simulink model "Copy_of_MPC_control"  (R2018a)
settings: Solver=FixedStepAuto  StartTime=0  StopTime=Tend  FixedStep=0.001  RelTol=5e-3
model workspace (MAT data in the model file):
  A_mu = 10
  B_reff = 8.386
  Cz = 7766.25
  DCT_Param : struct (value not decoded)
  D_reff = 0.25826
  Downshift_Speeds = [9.5625 12.9375 16.3125 19.6875 23.0625 26.4375 29.8125 33.1875 36.5625 39.9375 43.3125 46.6875 ... (28 elements, 4x7)]
  Pedal_Positions = [0.1 0.4 0.5 0.9]
  SUS : struct (value not decoded)
  Upshift_Speeds = [12.9375 16.3125 19.6875 33 26.4375 29.8125 33.1875 52.5 39.9375 43.3125 46.6875 77.25 ... (28 elements, 4x7)]
  VEH : struct (value not decoded)
  V_o = 16.7
  V_xlow = 1
  WH : struct (value not decoded)
  a = 1.4
  alpha_max = 1.5
  alpha_min = -1.5
  b = 1.8
  c_zo = 209651
  epsilon = 0.1
  h = 0.134
  path : struct (value not decoded)
  pio = 220000
  q_Fcx = 0
  q_Fz2 = 15.4
  q_Fzy = 0
  q_reo = 0.9974
  q_sx1 = -0.007764
  q_sx10 = 0.2824
  q_sx11 = 5.349
  q_sx12 = 0
  q_sx13 = 0
  q_sx14 = 0
  q_sx2 = 1.1915
  q_sx3 = 0.013948
  q_sx4 = 4.912
  q_sx5 = 1.02
  q_sx6 = 22.83
  q_sx7 = 0.7104
  q_sx8 = -0.023393
  q_sx9 = 0.6581
  q_sy1 = 0.00702
  q_sy2 = 0
  q_sy3 = 0.001515
  q_sy4 = 8.514e-05
  q_sy5 = 0
  q_sy6 = 0
  q_sy7 = 0.9008
  q_sy8 = -0.4089
  q_v1 = 0.0007742
  q_v2 = 0.04667
  r_Bx1 = 12.531
  r_Bx2 = 9.532
  r_Bx3 = 0
  r_By1 = 10.615
  r_By2 = 7.705
  r_By3 = 3.433e-06
  r_By4 = 0
  r_Cx1 = 1.019
  r_Cy1 = 1.0585
  r_Ex1 = -0.4487
  r_Ex2 = -0.4726
  r_Ey1 = 0.3132
  r_Ey2 = 7.63e-06
  r_Hx1 = 0.0002374
  r_Hy1 = 0.011646
  r_Hy2 = 7.63e-06
  r_Vy1 = 0.05654
  r_Vy2 = 7.63e-06
  r_Vy3 = 0
  r_Vy4 = 99.9
  r_Vy5 = 2
  r_Vy6 = 15.814
  r_o = 0.3135
  vehWidth = 2
  w = 1
symbols that are objects in the model workspace (value not decoded): VEH
undefined symbols (not defined in the file): C_Brake, C_Final, C_Front, C_Front_1, C_Front_2, C_Middle, C_out_Brake, C_out_Final, C_out_Front, C_out_Front_1, C_out_Front_2, C_out_Middle, Co, Cok_Brake, Cok_Final, Cok_Front_1, Cok_Front_2, Cok_Middle, Cso, D_out_Brake, D_out_Final, D_out_Front, D_out_Front_1, D_out_Front_2, D_out_Middle, Earlytochange, Earlytochange2, F, F_Brake, F_Final, F_Front, F_Front_1, F_Front_2, F_Middle, Fs, G_Brake, G_Final, G_Front_1, G_Front_2, G_Middle, G_sys_Brake, G_sys_Final, G_sys_Front, G_sys_Front_1, G_sys_Front_2, G_sys_Middle, Gd, Gd_Brake, Gd_Final, Gd_Front, Gd_Front_1, Gd_Front_2, Gd_Middle, Go, Gsd, Gso, H_Brake, H_Final, H_Front_1, H_Front_2 ... (+60)
libraries: simulink x10, sim3dlib x4, autolibutils x2, vehdynlibviscommon x2
(part 6 of 8)

== system Copy_of_MPC_control/all_system/Middle Observer2/Subsystem/Mpc_Simulator_Middle ==
  Vup : Inport  SampleTime=Ts  LockScale=on
  Yup : Inport  Port=2  SampleTime=Ts  LockScale=on
  Rs_V : Inport  Port=3  SampleTime=Ts  LockScale=on
  Rs : Inport  Port=4  SampleTime=Ts  LockScale=on
  Xh_sim : Inport  Port=5
  Clock : Clock
  Constant1 : Constant  Value=M  VectorParams1D=off  SampleTime=-1
  Constant2 : Constant  Value=Np  SampleTime=-1
  Constant3 : Constant  Value=Upd_flag  VectorParams1D=off  SampleTime=-1
  Constant4 : Constant  Value=Qc  VectorParams1D=off  SampleTime=-1
  Constant5 : Constant  Value=phi_Middle  VectorParams1D=off  SampleTime=-1
  Constant6 : Constant  Value=JE_Middle  VectorParams1D=off  SampleTime=-1
  Constant7 : Constant  Value=Upd_end  VectorParams1D=off  SampleTime=-1
  Constant8 : Constant  Value=Timetochange  VectorParams1D=off  SampleTime=-1
  F_Middle : Gain  Gain=F_Middle  Multiplication=Matrix(K*u) (u vector)
  MATLAB Function : MATLAB Function  TreatAsAtomicUnit=on  SystemSampleTime=Ts
  Unit Delay : UnitDelay  InitialCondition=[0;0]  SampleTime=Ts
  U : Outport
  Ref : Outport  Port=2
  wires:
  Unit Delay/1 -> MATLAB Function/15(u)
  MATLAB Function/2(U) -> Unit Delay/1, U/1
  MATLAB Function/1(Ref) -> Ref/1
  Xh_sim/1 -> F_Middle/1
  Constant4/1 -> MATLAB Function/7(Qc)
  Constant5/1 -> MATLAB Function/6(phi)
  Constant6/1 -> MATLAB Function/3(JE)
  Constant2/1 -> MATLAB Function/5(Np)
  Rs_V/1 -> MATLAB Function/12(Rs_V)
  Yup/1 -> MATLAB Function/9(Yup)
  Constant1/1 -> MATLAB Function/4(M)
  Clock/1 -> MATLAB Function/13(Tsim)
  F_Middle/1 -> MATLAB Function/8(Fxh)
  Vup/1 -> MATLAB Function/10(Vup)
  Rs/1 -> MATLAB Function/11(Rs)
  Constant3/1 -> MATLAB Function/1(Upd_flag)
  Constant7/1 -> MATLAB Function/14(Upd_end)
  Constant8/1 -> MATLAB Function/2(Timetochange)

== system Copy_of_MPC_control/all_system/Middle Observer2/Subsystem/Pose updete k ==
  XYplot_sim : Inport
  Velocity_sim : Inport  Port=2
  Heading_sim : Inport  Port=3
  Clock : Clock
  From Workspace : FromWorkspace  VariableName=Rs_V_now  SampleTime=Ts
  From Workspace1 : FromWorkspace  VariableName=Rs_Y_now  SampleTime=Ts
  From Workspace2 : FromWorkspace  VariableName=XYplot_X  SampleTime=Ts
  From Workspace3 : FromWorkspace  VariableName=XYplot_Y  SampleTime=Ts
  Mux : Mux  Inputs=2
  Reshape : Reshape  OutputDimensionality=Customize  OutputDimensions=[pick_num,2]
  Trajectroy : Constant  Value=XYplot  VectorParams1D=off  SampleTime=-1
  Unit Delay{,1..3} (4 alike) : UnitDelay  SampleTime=Ts
  Update : MATLAB Function  TreatAsAtomicUnit=on  SystemSampleTime=Ts
      settings: RTWFcnNameOpts=Use subsystem name
  Velocity_updated : Outport
  Heading_updated : Outport  Port=2
  wires:
  XYplot_sim/1 -> Update/5(XYplot_sim), Unit Delay3/1
  Heading_sim/1 -> Unit Delay2/1, Update/9(Heading_sim)
  Clock/1 -> Update/11(Tsim)
  Velocity_sim/1 -> Update/7(Velocity_sim), Unit Delay1/1
  Update/2(Heading_updated) -> Heading_updated/1
  Update/1(Velocity_updated) -> Velocity_updated/1
  From Workspace/1 -> Update/1(Rs_V_now)
  Update/3(Heading_end) -> Unit Delay/1
  Unit Delay/1 -> Update/12(Last_Heading_end)
  From Workspace1/1 -> Update/2(Rs_Y_now)
  Unit Delay1/1 -> Update/8(Last_Velocity_sim)
  Unit Delay2/1 -> Update/10(Last_Heading_sim)
  Unit Delay3/1 -> Update/6(Last_XYplot_sim)
  Mux/1 -> Reshape/1
  From Workspace2/1 -> Mux/1
  From Workspace3/1 -> Mux/2
  Trajectroy/1 -> Update/3(XYline)
  Reshape/1 -> Update/4(XYplot)

== system Copy_of_MPC_control/all_system/Middle Observer2/Subsystem/VH2P ==
  Velocities : Inport
  HeadingAngles : Inport  Port=2
  Initial position : Inport  Port=3
  Iintial Velocities : Inport  Port=4
  Iintial HeadingAngles : Inport  Port=5
  Tsim : Inport  Port=6
  LastTsim : Inport  Port=7
  Resettable Delay : Delay  DelayLength=1  InitialConditionSource=Input port  SampleTime=Ts
      settings: InputPortMap=u0,p4
  Resettable Delay1 : Delay  DelayLength=1  InitialConditionSource=Input port  SampleTime=Ts
      settings: InputPortMap=u0,p4
  Resettable Delay2 : Delay  DelayLength=1  InitialConditionSource=Input port  SampleTime=Ts
      settings: InputPortMap=u0,p4
  YV2P : MATLAB Function  TreatAsAtomicUnit=on  SystemSampleTime=Ts
  Position : Outport
  wires:
  YV2P/1(Position) -> Resettable Delay/1, Position/1
  LastTsim/1 -> YV2P/6(LastTsim)
  Velocities/1 -> Resettable Delay1/1, YV2P/1(Velocity)
  Resettable Delay1/1 -> YV2P/3(LastVelocity)
  HeadingAngles/1 -> YV2P/2(Yaw), Resettable Delay2/1
  Resettable Delay2/1 -> YV2P/4(LastYaw)
  Resettable Delay/1 -> YV2P/7(Lastpostion)
  Initial position/1 -> Resettable Delay/2
  Iintial Velocities/1 -> Resettable Delay1/2
  Iintial HeadingAngles/1 -> Resettable Delay2/2
  Tsim/1 -> YV2P/5(Tsim)

== system Copy_of_MPC_control/all_system/Middle Observer2/Subsystem/YV_update_Np ==
  XY_sim : Inport
  Velocity_sim : Inport  Port=2
  Heading_sim : Inport  Port=3
  From Workspace1 : FromWorkspace  VariableName=T_sim  SampleTime=Ts
  From Workspace3 : FromWorkspace  VariableName=XY_Ref_Upd  SampleTime=Ts
  MATLAB Function2 : MATLAB Function  TreatAsAtomicUnit=on  SystemSampleTime=Ts
  Unit Delay1 : UnitDelay  SampleTime=Ts
  Unit Delay4 : UnitDelay  SampleTime=Ts
  Unit Delay5 : UnitDelay  SampleTime=Ts
  Velocity : Outport
  Heading angle : Outport  Port=2
  wires:
  MATLAB Function2/1(Velocity_updated) -> Velocity/1
  From Workspace3/1 -> MATLAB Function2/1(XY_ref)
  MATLAB Function2/2(Heading_updated) -> Heading angle/1
  From Workspace1/1 -> MATLAB Function2/8(Tsim)
  XY_sim/1 -> Unit Delay1/1, MATLAB Function2/2(XY_sim)
  Velocity_sim/1 -> MATLAB Function2/4(Velocity_sim), Unit Delay5/1
  Heading_sim/1 -> MATLAB Function2/6(Yaw_sim), Unit Delay4/1
  Unit Delay1/1 -> MATLAB Function2/3(LastXY_sim)
  Unit Delay5/1 -> MATLAB Function2/5(LastVelocity_sim)
  Unit Delay4/1 -> MATLAB Function2/7(LastYaw_sim)

== system Copy_of_MPC_control/all_system/Middle_simulator1/VH2P/Trigger ==
  Clock9 : Clock
  Constant1 : Constant  Value=Timetochange
  Trigger : MATLAB Function  TreatAsAtomicUnit=on
  Trig : Outport
  wires:
  Constant1/1 -> Trigger/2(Timetochange)
  Clock9/1 -> Trigger/1(timing)
  Trigger/1(Trigger) -> Trig/1

== system Copy_of_MPC_control/all_system/Visualization1/3D Engine/3D Engine ==
  VehFdbk : Inport
  3D Body Offset : Constant  Value=single(0.0112)  OutDataTypeStr=single
  Add1 : Sum  Inputs=-+
  Add3 : Sum  Inputs=-+-
  Bus Selector : BusSelector  OutputSignals=Body.X,Body.Y,Body.Z,Body.phi,Body.theta,Body.psi
  Bus Selector2 : BusSelector  OutputSignals=Wheels.zAxle,Wheels.omega,Driveline.WhlAng
  Bus Selector3 : BusSelector  OutputSignals=Body.ZHP
  Constant1 : Constant  Value=zeros(4,1)  OutDataTypeStr=single
  Constant2 : Constant  Value=0  OutDataTypeStr=single
  Constant8 : Constant  Value=h
  Data Type Conversion{1,4..10,12} (9 alike) : DataTypeConversion  OutDataTypeStr=single
  Demux{,1..3} (4 alike) : Demux
  Integrator : Integrator  WrapState=on  WrappedStateUpperValue=2*pi  WrappedStateLowerValue=0  ZeroCross=off
  Part Rotation Concatenation : Subsystem
  Part Translation Concatenation : Subsystem
  Rate Transition : RateTransition  OutPortSampleTime=dt3D
  Scale : Subsystem
  Simulation 3D Engine 1 : sim3dlib/Simulation 3D Config  Priority=1  ProjectFormat=Executable  ProjectName=VehicleSimulation.exe  SceneDesc=Straight road  OpVisEn=off  Ts=dt3D
      settings: AttributesFormatString=Priority: %<Priority>
  Unary Minus : UnaryMinus
  Vehicle Actor Transform Set : sim3dlib/Simulation 3D Actor Transform Set  ActorTag=SimulinkVehicle1  ActorType=Passenger vehicle  PassVehMesh=Muscle car  VehColor=Red  NumberOfParts=5  CustNumOfParts=3  Translation=[0 0 1; 0 0 0; 0 0 0; 0 0 0; 0 0 0]  Rotation=[0 0 0; 0 0 0; 0 0 0; 0 0 0; 0 0 0]  Scale=[1 1 1; 1 1 1; 1 1 1; 1 1 1; 1 1 1]  Ts=dt3D
  wires:
  Unary Minus/1 -> Integrator/1
  Bus Selector3/1 -> Add3/2  "<ZHP>"
  Add3/1 -> Data Type Conversion12/1
  Bus Selector2/1 -> Add3/3  "<zAxle>"
  Constant8/1 -> Add3/1
  Rate Transition/1 -> Bus Selector/1, Bus Selector3/1, Bus Selector2/1
  Scale/1(ScaleOut) -> Vehicle Actor Transform Set/3
  Demux/4 -> Part Rotation Concatenation/7(WheelRearRight Ptich)
  Demux/3 -> Part Rotation Concatenation/6(WheelRearLeft Pitch)
  Demux/2 -> Part Rotation Concatenation/5(WheelFrontRight Pitch)
  Demux/1 -> Part Rotation Concatenation/4(WheelFrontLeft Pitch)
  Constant1/1 -> Demux2/1
  Bus Selector/4 -> Data Type Conversion7/1  "<phi>"
  Data Type Conversion6/1 -> Add1/1
  Part Rotation Concatenation/1(ConcatOut) -> Vehicle Actor Transform Set/2
  Part Translation Concatenation/1(ConcatOut) -> Vehicle Actor Transform Set/1
  Data Type Conversion12/1 -> Demux3/1
  Demux3/4 -> Part Translation Concatenation/15(WheelRearRightZ)
  Demux3/3 -> Part Translation Concatenation/14(WheelRearLeftZ)
  Demux3/1 -> Part Translation Concatenation/12(WheelFrontLeftZ)
  Demux3/2 -> Part Translation Concatenation/13(WheelFrontRightZ)
  VehFdbk/1 -> Rate Transition/1
  Add1/1 -> Part Translation Concatenation/3(BodyZ)
  3D Body Offset/1 -> Add1/2
  Demux1/4 -> Part Rotation Concatenation/15(WheelRearRight Yaw)
  Demux1/3 -> Part Rotation Concatenation/14(WheelRearLeft Yaw)
  Demux2/1 -> Part Rotation Concatenation/8(WheelFrontLeft Roll)
  Demux2/2 -> Part Rotation Concatenation/9(WheelFrontRight Roll)
  Demux2/3 -> Part Rotation Concatenation/10(WheelRearLeft Roll)
  Demux2/4 -> Part Rotation Concatenation/11(WheelRearRight Roll)
  Bus Selector2/3 -> Data Type Conversion9/1  "<WhlAng>"
  Bus Selector2/2 -> Unary Minus/1  "<omega>"
  Data Type Conversion9/1 -> Demux1/1
  Demux1/1 -> Part Rotation Concatenation/12(WheelFrontLeft Yaw)
  Demux1/2 -> Part Rotation Concatenation/13(WheelFrontRight Yaw)
  Integrator/1 -> Data Type Conversion1/1
  Data Type Conversion1/1 -> Demux/1
  Data Type Conversion8/1 -> Part Rotation Concatenation/2(Body Ptich)
  Data Type Conversion5/1 -> Part Translation Concatenation/2(BodyY)
  Data Type Conversion10/1 -> Part Rotation Concatenation/3(Body Yaw)
  Constant2/1 -> Part Translation Concatenation/5(WheelFrontRightX), Part Translation Concatenation/6(WheelRearLeftX), Part Translation Concatenation/7(WheelRearRightX), Part Translation Concatenation/8(WheelFrontLeftY), Part Translation Concatenation/9(WheelFrontRightY), Part Translation Concatenation/10(WheelRearLeftY), Part Translation Concatenation/11(WheelRearRightY), Part Translation Concatenation/4(WheelFrontLeftX)
  Data Type Conversion4/1 -> Part Translation Concatenation/1(BodyX)
  Data Type Conversion7/1 -> Part Rotation Concatenation/1(Body Roll)
  Bus Selector/1 -> Data Type Conversion4/1  "<X>"
  Bus Selector/2 -> Data Type Conversion5/1  "<Y>"
  Bus Selector/3 -> Data Type Conversion6/1  "<Z>"
  Bus Selector/6 -> Data Type Conversion10/1  "<psi>"
  Bus Selector/5 -> Data Type Conversion8/1  "<theta>"

== system Copy_of_MPC_control/all_system/Visualization1/3D Engine/3D Engine Disabled ==
  VehFdbk : Inport
  Terminator : Terminator
  wires:
  VehFdbk/1 -> Terminator/1

== system Copy_of_MPC_control/observer123/Final Observer2/Subsystem/Mpc_Simulator_Final ==
  Vup : Inport  SampleTime=Ts  LockScale=on
  Yup : Inport  Port=2  SampleTime=Ts  LockScale=on
  Rs_V : Inport  Port=3  SampleTime=Ts  LockScale=on
  Rs : Inport  Port=4  SampleTime=Ts  LockScale=on
  Xh_sim : Inport  Port=5
  Clock : Clock
  Constant1 : Constant  Value=M  VectorParams1D=off  SampleTime=-1
  Constant2 : Constant  Value=Np  SampleTime=-1
  Constant3 : Constant  Value=Upd_flag  VectorParams1D=off  SampleTime=-1
  Constant4 : Constant  Value=Qc  VectorParams1D=off  SampleTime=-1
  Constant5 : Constant  Value=phi_Final  VectorParams1D=off  SampleTime=-1
  Constant6 : Constant  Value=JE_Final  VectorParams1D=off  SampleTime=-1
  Constant7 : Constant  Value=Upd_end  VectorParams1D=off  SampleTime=-1
  Constant8 : Constant  Value=Timetochange  VectorParams1D=off  SampleTime=-1
  F_Final : Gain  Gain=F_Final  Multiplication=Matrix(K*u) (u vector)
  MATLAB Function : MATLAB Function  TreatAsAtomicUnit=on  SystemSampleTime=Ts
  Unit Delay : UnitDelay  InitialCondition=[0;0]  SampleTime=Ts
  U : Outport
  Ref : Outport  Port=2
  wires:
  Unit Delay/1 -> MATLAB Function/15(u)
  MATLAB Function/2(U) -> Unit Delay/1, U/1
  MATLAB Function/1(Ref) -> Ref/1
  Xh_sim/1 -> F_Final/1
  Constant4/1 -> MATLAB Function/7(Qc)
  Constant5/1 -> MATLAB Function/6(phi)
  Constant6/1 -> MATLAB Function/3(JE)
  Constant2/1 -> MATLAB Function/5(Np)
  Rs_V/1 -> MATLAB Function/12(Rs_V)
  Yup/1 -> MATLAB Function/9(Yup)
  Constant1/1 -> MATLAB Function/4(M)
  Clock/1 -> MATLAB Function/13(Tsim)
  F_Final/1 -> MATLAB Function/8(Fxh)
  Vup/1 -> MATLAB Function/10(Vup)
  Rs/1 -> MATLAB Function/11(Rs)
  Constant3/1 -> MATLAB Function/1(Upd_flag)
  Constant7/1 -> MATLAB Function/14(Upd_end)
  Constant8/1 -> MATLAB Function/2(Timetochange)

== system Copy_of_MPC_control/observer123/Final Observer2/Subsystem/Pose updete k ==
  XYplot_sim : Inport
  Velocity_sim : Inport  Port=2
  Heading_sim : Inport  Port=3
  Clock : Clock
  From Workspace : FromWorkspace  VariableName=Rs_V_now  SampleTime=Ts
  From Workspace1 : FromWorkspace  VariableName=Rs_Y_now  SampleTime=Ts
  From Workspace2 : FromWorkspace  VariableName=XYplot_X  SampleTime=Ts
  From Workspace3 : FromWorkspace  VariableName=XYplot_Y  SampleTime=Ts
  Mux : Mux  Inputs=2
  Reshape : Reshape  OutputDimensionality=Customize  OutputDimensions=[pick_num,2]
  Trajectroy : Constant  Value=XYplot  VectorParams1D=off  SampleTime=-1
  Unit Delay{,1..3} (4 alike) : UnitDelay  SampleTime=Ts
  Update : MATLAB Function  TreatAsAtomicUnit=on  SystemSampleTime=Ts
      settings: RTWFcnNameOpts=Use subsystem name
  Velocity_updated : Outport
  Heading_updated : Outport  Port=2
  wires:
  XYplot_sim/1 -> Update/5(XYplot_sim), Unit Delay3/1
  Heading_sim/1 -> Unit Delay2/1, Update/9(Heading_sim)
  Clock/1 -> Update/11(Tsim)
  Velocity_sim/1 -> Update/7(Velocity_sim), Unit Delay1/1
  Update/2(Heading_updated) -> Heading_updated/1
  Update/1(Velocity_updated) -> Velocity_updated/1
  From Workspace/1 -> Update/1(Rs_V_now)
  Update/3(Heading_end) -> Unit Delay/1
  Unit Delay/1 -> Update/12(Last_Heading_end)
  From Workspace1/1 -> Update/2(Rs_Y_now)
  Unit Delay1/1 -> Update/8(Last_Velocity_sim)
  Unit Delay2/1 -> Update/10(Last_Heading_sim)
  Unit Delay3/1 -> Update/6(Last_XYplot_sim)
  Mux/1 -> Reshape/1
  From Workspace2/1 -> Mux/1
  From Workspace3/1 -> Mux/2
  Trajectroy/1 -> Update/3(XYline)
  Reshape/1 -> Update/4(XYplot)

== system Copy_of_MPC_control/observer123/Final Observer2/Subsystem/VH2P ==
  Velocities : Inport
  HeadingAngles : Inport  Port=2
  Initial position : Inport  Port=3
  Iintial Velocities : Inport  Port=4
  Iintial HeadingAngles : Inport  Port=5
  Tsim : Inport  Port=6
  LastTsim : Inport  Port=7
  Initial trigger : Inport  Port=8
  Initial trigger1 : InportShadow  Port=8
  Initial trigger2 : InportShadow  Port=8
  Resettable Delay : Delay  DelayLength=1  InitialConditionSource=Input port  ExternalReset=Falling  SampleTime=Ts
      settings: InputPortMap=u0,r5,p4
  Resettable Delay1 : Delay  DelayLength=1  InitialConditionSource=Input port  ExternalReset=Falling  SampleTime=Ts
      settings: InputPortMap=u0,r5,p4
  Resettable Delay2 : Delay  DelayLength=1  InitialConditionSource=Input port  ExternalReset=Falling  SampleTime=Ts
      settings: InputPortMap=u0,r5,p4
  YV2P : MATLAB Function  TreatAsAtomicUnit=on  SystemSampleTime=Ts
  Position : Outport
  wires:
  YV2P/1(Position) -> Resettable Delay/1, Position/1
  LastTsim/1 -> YV2P/6(LastTsim)
  Velocities/1 -> Resettable Delay1/1, YV2P/1(Velocity)
  Resettable Delay1/1 -> YV2P/3(LastVelocity)
  HeadingAngles/1 -> YV2P/2(Yaw), Resettable Delay2/1
  Resettable Delay2/1 -> YV2P/4(LastYaw)
  Resettable Delay/1 -> YV2P/7(Lastpostion)
  Initial position/1 -> Resettable Delay/3
  Iintial Velocities/1 -> Resettable Delay1/3
  Iintial HeadingAngles/1 -> Resettable Delay2/3
  Tsim/1 -> YV2P/5(Tsim)
  Initial trigger/1 -> Resettable Delay/2
  Initial trigger1/1 -> Resettable Delay1/2
  Initial trigger2/1 -> Resettable Delay2/2

== system Copy_of_MPC_control/observer123/Final Observer2/Subsystem/YV_update_Np ==
  XY_sim : Inport
  Velocity_sim : Inport  Port=2
  Heading_sim : Inport  Port=3
  From Workspace1 : FromWorkspace  VariableName=T_sim  SampleTime=Ts
  From Workspace3 : FromWorkspace  VariableName=XY_Ref_Upd  SampleTime=Ts
  MATLAB Function2 : MATLAB Function  TreatAsAtomicUnit=on  SystemSampleTime=Ts
  Unit Delay1 : UnitDelay  SampleTime=Ts
  Unit Delay4 : UnitDelay  SampleTime=Ts
  Unit Delay5 : UnitDelay  SampleTime=Ts
  Velocity : Outport
  Heading angle : Outport  Port=2
  wires:
  MATLAB Function2/1(Velocity_updated) -> Velocity/1
  From Workspace3/1 -> MATLAB Function2/1(XY_ref)
  MATLAB Function2/2(Heading_updated) -> Heading angle/1
  From Workspace1/1 -> MATLAB Function2/8(Tsim)
  XY_sim/1 -> Unit Delay1/1, MATLAB Function2/2(XY_sim)
  Velocity_sim/1 -> MATLAB Function2/4(Velocity_sim), Unit Delay5/1
  Heading_sim/1 -> MATLAB Function2/6(Yaw_sim), Unit Delay4/1
  Unit Delay1/1 -> MATLAB Function2/3(LastXY_sim)
  Unit Delay5/1 -> MATLAB Function2/5(LastVelocity_sim)
  Unit Delay4/1 -> MATLAB Function2/7(LastYaw_sim)

== system Copy_of_MPC_control/observer123/Middle Observer2/Subsystem/Mpc_Simulator_Middle ==
  Vup : Inport  SampleTime=Ts  LockScale=on
  Yup : Inport  Port=2  SampleTime=Ts  LockScale=on
  Rs_V : Inport  Port=3  SampleTime=Ts  LockScale=on
  Rs : Inport  Port=4  SampleTime=Ts  LockScale=on
  Xh_sim : Inport  Port=5
  Clock : Clock
  Constant1 : Constant  Value=M  VectorParams1D=off  SampleTime=-1
  Constant2 : Constant  Value=Np  SampleTime=-1
  Constant3 : Constant  Value=Upd_flag  VectorParams1D=off  SampleTime=-1
  Constant4 : Constant  Value=Qc  VectorParams1D=off  SampleTime=-1
  Constant5 : Constant  Value=phi_Middle  VectorParams1D=off  SampleTime=-1
  Constant6 : Constant  Value=JE_Middle  VectorParams1D=off  SampleTime=-1
  Constant7 : Constant  Value=Upd_end  VectorParams1D=off  SampleTime=-1
  Constant8 : Constant  Value=Timetochange  VectorParams1D=off  SampleTime=-1
  F_Middle : Gain  Gain=F_Middle  Multiplication=Matrix(K*u) (u vector)
  MATLAB Function : MATLAB Function  TreatAsAtomicUnit=on  SystemSampleTime=Ts
  Unit Delay : UnitDelay  InitialCondition=[0;0]  SampleTime=Ts
  U : Outport
  Ref : Outport  Port=2
  wires:
  Unit Delay/1 -> MATLAB Function/15(u)
  MATLAB Function/2(U) -> Unit Delay/1, U/1
  MATLAB Function/1(Ref) -> Ref/1
  Xh_sim/1 -> F_Middle/1
  Constant4/1 -> MATLAB Function/7(Qc)
  Constant5/1 -> MATLAB Function/6(phi)
  Constant6/1 -> MATLAB Function/3(JE)
  Constant2/1 -> MATLAB Function/5(Np)
  Rs_V/1 -> MATLAB Function/12(Rs_V)
  Yup/1 -> MATLAB Function/9(Yup)
  Constant1/1 -> MATLAB Function/4(M)
  Clock/1 -> MATLAB Function/13(Tsim)
  F_Middle/1 -> MATLAB Function/8(Fxh)
  Vup/1 -> MATLAB Function/10(Vup)
  Rs/1 -> MATLAB Function/11(Rs)
  Constant3/1 -> MATLAB Function/1(Upd_flag)
  Constant7/1 -> MATLAB Function/14(Upd_end)
  Constant8/1 -> MATLAB Function/2(Timetochange)

== system Copy_of_MPC_control/observer123/Middle Observer2/Subsystem/Pose updete k ==
  XYplot_sim : Inport
  Velocity_sim : Inport  Port=2
  Heading_sim : Inport  Port=3
  Clock : Clock
  From Workspace : FromWorkspace  VariableName=Rs_V_now  SampleTime=Ts
  From Workspace1 : FromWorkspace  VariableName=Rs_Y_now  SampleTime=Ts
  From Workspace2 : FromWorkspace  VariableName=XYplot_X  SampleTime=Ts
  From Workspace3 : FromWorkspace  VariableName=XYplot_Y  SampleTime=Ts
  Mux : Mux  Inputs=2
  Reshape : Reshape  OutputDimensionality=Customize  OutputDimensions=[pick_num,2]
  Trajectroy : Constant  Value=XYplot  VectorParams1D=off  SampleTime=-1
  Unit Delay{,1..3} (4 alike) : UnitDelay  SampleTime=Ts
  Update : MATLAB Function  TreatAsAtomicUnit=on  SystemSampleTime=Ts
      settings: RTWFcnNameOpts=Use subsystem name
  Velocity_updated : Outport
  Heading_updated : Outport  Port=2
  wires:
  XYplot_sim/1 -> Update/5(XYplot_sim), Unit Delay3/1
  Heading_sim/1 -> Unit Delay2/1, Update/9(Heading_sim)
  Clock/1 -> Update/11(Tsim)
  Velocity_sim/1 -> Update/7(Velocity_sim), Unit Delay1/1
  Update/2(Heading_updated) -> Heading_updated/1
  Update/1(Velocity_updated) -> Velocity_updated/1
  From Workspace/1 -> Update/1(Rs_V_now)
  Update/3(Heading_end) -> Unit Delay/1
  Unit Delay/1 -> Update/12(Last_Heading_end)
  From Workspace1/1 -> Update/2(Rs_Y_now)
  Unit Delay1/1 -> Update/8(Last_Velocity_sim)
  Unit Delay2/1 -> Update/10(Last_Heading_sim)
  Unit Delay3/1 -> Update/6(Last_XYplot_sim)
  Mux/1 -> Reshape/1
  From Workspace2/1 -> Mux/1
  From Workspace3/1 -> Mux/2
  Trajectroy/1 -> Update/3(XYline)
  Reshape/1 -> Update/4(XYplot)

== system Copy_of_MPC_control/observer123/Middle Observer2/Subsystem/VH2P ==
  Velocities : Inport
  HeadingAngles : Inport  Port=2
  Initial position : Inport  Port=3
  Iintial Velocities : Inport  Port=4
  Iintial HeadingAngles : Inport  Port=5
  Tsim : Inport  Port=6
  LastTsim : Inport  Port=7
  Resettable Delay : Delay  DelayLength=1  InitialConditionSource=Input port  SampleTime=Ts
      settings: InputPortMap=u0,p4
  Resettable Delay1 : Delay  DelayLength=1  InitialConditionSource=Input port  SampleTime=Ts
      settings: InputPortMap=u0,p4
  Resettable Delay2 : Delay  DelayLength=1  InitialConditionSource=Input port  SampleTime=Ts
      settings: InputPortMap=u0,p4
  YV2P : MATLAB Function  TreatAsAtomicUnit=on  SystemSampleTime=Ts
  Position : Outport
  wires:
  YV2P/1(Position) -> Resettable Delay/1, Position/1
  LastTsim/1 -> YV2P/6(LastTsim)
  Velocities/1 -> Resettable Delay1/1, YV2P/1(Velocity)
  Resettable Delay1/1 -> YV2P/3(LastVelocity)
  HeadingAngles/1 -> YV2P/2(Yaw), Resettable Delay2/1
  Resettable Delay2/1 -> YV2P/4(LastYaw)
  Resettable Delay/1 -> YV2P/7(Lastpostion)
  Initial position/1 -> Resettable Delay/2
  Iintial Velocities/1 -> Resettable Delay1/2
  Iintial HeadingAngles/1 -> Resettable Delay2/2
  Tsim/1 -> YV2P/5(Tsim)

== system Copy_of_MPC_control/observer123/Middle Observer2/Subsystem/YV_update_Np ==
  XY_sim : Inport
  Velocity_sim : Inport  Port=2
  Heading_sim : Inport  Port=3
  From Workspace1 : FromWorkspace  VariableName=T_sim  SampleTime=Ts
  From Workspace3 : FromWorkspace  VariableName=XY_Ref_Upd  SampleTime=Ts
  MATLAB Function2 : MATLAB Function  TreatAsAtomicUnit=on  SystemSampleTime=Ts
  Unit Delay1 : UnitDelay  SampleTime=Ts
  Unit Delay4 : UnitDelay  SampleTime=Ts
  Unit Delay5 : UnitDelay  SampleTime=Ts
  Velocity : Outport
  Heading angle : Outport  Port=2
  wires:
  MATLAB Function2/1(Velocity_updated) -> Velocity/1
  From Workspace3/1 -> MATLAB Function2/1(XY_ref)
  MATLAB Function2/2(Heading_updated) -> Heading angle/1
  From Workspace1/1 -> MATLAB Function2/8(Tsim)
  XY_sim/1 -> Unit Delay1/1, MATLAB Function2/2(XY_sim)
  Velocity_sim/1 -> MATLAB Function2/4(Velocity_sim), Unit Delay5/1
  Heading_sim/1 -> MATLAB Function2/6(Yaw_sim), Unit Delay4/1
  Unit Delay1/1 -> MATLAB Function2/3(LastXY_sim)
  Unit Delay5/1 -> MATLAB Function2/5(LastVelocity_sim)
  Unit Delay4/1 -> MATLAB Function2/7(LastYaw_sim)

== system Copy_of_MPC_control/Controllers/Brake Controller/Brake Pressure Control/Bang Bang ABS/Bang-bang controller ==
  in_1 : Inport
  Constant : Constant  Value=0
  Data Type Conversion1 : DataTypeConversion  OutDataTypeStr=double  SaturateOnIntegerOverflow=on  RndMeth=Zero
  Data Type Conversion2 : DataTypeConversion  OutDataTypeStr=double  SaturateOnIntegerOverflow=on  RndMeth=Zero
  Relational Operator : RelationalOperator  Operator=>  OutDataTypeStr=boolean  RndMeth=Nearest  InputSameDT=on
  Relational Operator1 : RelationalOperator  Operator=<  OutDataTypeStr=boolean  RndMeth=Nearest  InputSameDT=on
  Sum : Sum  Inputs=+-  SaturateOnIntegerOverflow=on  InputSameDT=on  OutDataTypeStr=Inherit: Same as first input
  out_1 : Outport  InitialOutput=0
  wires:
  Data Type Conversion2/1 -> Sum/2
  Data Type Conversion1/1 -> Sum/1
  Sum/1 -> out_1/1
  Relational Operator/1 -> Data Type Conversion1/1
  Relational Operator1/1 -> Data Type Conversion2/1
  Constant/1 -> Relational Operator/2, Relational Operator1/2
  in_1/1 -> Relational Operator1/1, Relational Operator/1

== system Copy_of_MPC_control/Visualization/3D Engine/3D Engine/Scale/PartConcatenation ==
  BodyX : Inport
  BodyY : Inport  Port=2
  BodyZ : Inport  Port=3
  WheelFrontLeftX : Inport  Port=4
  WheelFrontLeftY : Inport  Port=5
  WheelFrontLeftZ : Inport  Port=6
  WheelFrontRightX : Inport  Port=7
  WheelFrontRightY : Inport  Port=8
  WheelFrontRightZ : Inport  Port=9
  WheelRearLeftX : Inport  Port=10
  WheelRearLeftY : Inport  Port=11
  WheelRearLeftZ : Inport  Port=12
  WheelRearRightX : Inport  Port=13
  WheelRearRightY : Inport  Port=14
  WheelRearRightZ : Inport  Port=15
  AllParts : Concatenate  NumInputs=5  Mode=Multidimensional array
  Body : Concatenate  NumInputs=3  Mode=Multidimensional array  ConcatenateDimension=2
  WheelFrontLeft : Concatenate  NumInputs=3  Mode=Multidimensional array  ConcatenateDimension=2
  WheelFrontRight : Concatenate  NumInputs=3  Mode=Multidimensional array  ConcatenateDimension=2
  WheelRearLeft : Concatenate  NumInputs=3  Mode=Multidimensional array  ConcatenateDimension=2
  WheelRearRight : Concatenate  NumInputs=3  Mode=Multidimensional array  ConcatenateDimension=2
  ConcatOut : Outport
  wires:
  BodyX/1 -> Body/1
  BodyZ/1 -> Body/3
  WheelFrontLeftX/1 -> WheelFrontLeft/1
  WheelFrontLeftZ/1 -> WheelFrontLeft/3
  WheelFrontLeftY/1 -> WheelFrontLeft/2
  BodyY/1 -> Body/2
  WheelFrontLeft/1 -> AllParts/2
  WheelRearRightX/1 -> WheelRearRight/1
  Body/1 -> AllParts/1
  WheelRearLeft/1 -> AllParts/4
  WheelFrontRight/1 -> AllParts/3
  WheelRearRightZ/1 -> WheelRearRight/3
  WheelFrontRightY/1 -> WheelFrontRight/2
  WheelFrontRightX/1 -> WheelFrontRight/1
  WheelRearRightY/1 -> WheelRearRight/2
  WheelRearLeftZ/1 -> WheelRearLeft/3
  AllParts/1 -> ConcatOut/1
  WheelRearLeftY/1 -> WheelRearLeft/2
  WheelRearRight/1 -> AllParts/5
  WheelRearLeftX/1 -> WheelRearLeft/1
  WheelFrontRightZ/1 -> WheelFrontRight/3

== system Copy_of_MPC_control/all_system/Controllers1/Brake Controller/Brake Pressure Control/Bang Bang ABS ==
  Pref : Inport
  xdot : Inport  Port=2
  <Kappa> : Inport  Port=3
  Abs : Abs
  Add : Sum  Inputs=-+
  Bang-bang controller : Subsystem  mask(Sign){}
      mask help: y = sign(x)
      mask Help: Sign Function:\n\t\t\ty = 1 if x > 0\n\t\t\ty = 0 if x = 0\n\t\t\ty = -1 if x < 0
      mask Display: plot(-50,-50,50,50,[-50,50],[0,0],[0,0],[-50,50],[-40,0],[-30,-30],[0,40],[30,30])
  Compare To Constant : simulink/Logic and Bit Operations/Compare To Constant  relop=>=  const=.2  OutDataTypeStr=boolean
  Compare To Constant1 : simulink/Logic and Bit Operations/Compare To Constant  relop=>=  const=.75  OutDataTypeStr=boolean
  Compare To Constant2 : simulink/Logic and Bit Operations/Compare To Constant  relop=>=  const=.5  OutDataTypeStr=boolean
  Constant : Constant  Value=.25
  Debounce : autolibutils/Debounce  DbcOn_Cnts=.1*.001  DbcOff_Cnts=.1*.001  aMode=aMode
      settings: SourceProductName=Powertrain Blockset  SourceProductBaseCode=PW
  Gain : Gain  Gain=200
  Logical Operator : Logic  Inputs=3  AllPortsSameDT=off  OutDataTypeStr=boolean
  Rate Transition : RateTransition  OutPortSampleTime=.001
  Rate Transition1 : RateTransition
  Switch : Switch  Criteria=u2 > Threshold  ZeroCross=off
  PCmd : Outport
  wires:
  Bang-bang controller/1(out_1) -> Gain/1
  Add/1 -> Bang-bang controller/1(in_1)
  Rate Transition1/1 -> PCmd/1
  <Kappa>/1 -> Rate Transition/1
  Pref/1 -> Switch/3, Compare To Constant1/1  "Pref"
  Constant/1 -> Add/2  "slip ref"
  Switch/1 -> Rate Transition1/1
  Rate Transition/1 -> Add/1, Compare To Constant/1
  Logical Operator/1 -> Debounce/1
  Compare To Constant/1 -> Logical Operator/2
  Compare To Constant1/1 -> Logical Operator/3
  Debounce/1 -> Switch/2
  xdot/1 -> Abs/1
  Abs/1 -> Compare To Constant2/1
  Compare To Constant2/1 -> Logical Operator/1
  Gain/1 -> Switch/1

== system Copy_of_MPC_control/all_system/Controllers1/Brake Controller/Brake Pressure Control/Open Loop ==
  Pref : Inport
  PCmd : Outport
  wires:
  Pref/1 -> PCmd/1  "Reference Slip"

== system Copy_of_MPC_control/all_system/Controllers1/Transmission Controller/TCM/Neutral Select ==
  AccCmd : Inport
  EngSpd : Inport  Port=2
  Constant : Constant  Value=1200
  Constant1 : Constant  Value=1e-6
  Logical Operator : Logic  AllPortsSameDT=off  OutDataTypeStr=boolean
  Relational Operator : RelationalOperator  Operator=<=  OutDataTypeStr=boolean  RndMeth=Simplest
  Relational Operator1 : RelationalOperator  Operator=<=  OutDataTypeStr=boolean  RndMeth=Simplest
  Saturation1 : Saturate  UpperLimit=10e3  LowerLimit=0
  rad/s to RPM : Gain  Gain=30/pi
  Neutral Select : Outport
  wires:
  Saturation1/1 -> Relational Operator/1
  Relational Operator1/1 -> Logical Operator/1
  AccCmd/1 -> Relational Operator1/1
  Constant1/1 -> Relational Operator1/2
  Logical Operator/1 -> Neutral Select/1
  Constant/1 -> Relational Operator/2
  Relational Operator/1 -> Logical Operator/2
  rad/s to RPM/1 -> Saturation1/1
  EngSpd/1 -> rad/s to RPM/1

== system Copy_of_MPC_control/all_system/Controllers1/Transmission Controller/TCM/TCM Shift Controller/calc ==
  note: Determine if next gear will be
      | higher or lower than current gear
  gear : Inport
  pedal : Inport  Port=2
  speed : Inport  Port=3
  f : TriggerPort  TriggerType=function-call  VariantControl=Variant  StatesWhenEnabling=reset
      settings: CopyFcn=Stateflow.SLINSF.SimulinkMan.removeBlockPreDeleteFcn  PreDeleteFcn=Stateflow.SLINSF.SimulinkMan.unsafePredeleteFcn
  Add1 : Sum  Inputs=+-
  Add3 : Sum  Inputs=+-
  Add4 : Sum  Inputs=+-
  Calculate Upshift Threshold : Lookup_n-D  BreakpointsForDimension1=Pedal_Positions  BreakpointsForDimension2=1:7  Table=Upshift_Speeds  ExtrapMethod=Clip  UseLastTableValue=on  InternalRulePriority=Speed  RndMeth=Simplest  InputSameDT=on
  Calculate Downshift Threshold : Lookup_n-D  BreakpointsForDimension1=Pedal_Positions  BreakpointsForDimension2=2:8  Table=Downshift_Speeds  ExtrapMethod=Clip  UseLastTableValue=on  InternalRulePriority=Speed  RndMeth=Simplest  InputSameDT=on
  SpdThr : Outport
  wires:
  pedal/1 -> Calculate Downshift Threshold/1, Calculate Upshift Threshold/1
  gear/1 -> Calculate Downshift Threshold/2, Calculate Upshift Threshold/2
  Calculate Downshift Threshold/1 -> Add3/2
  Calculate Upshift Threshold/1 -> Add1/1
  speed/1 -> Add1/2, Add3/1
  Add1/1 -> Add4/1
  Add3/1 -> Add4/2
  Add4/1 -> SpdThr/1

== system Copy_of_MPC_control/all_system/Controllers1/Transmission Controller/TCM/TCM Shift Controller/calc_down ==
  gear : Inport
  pedal : Inport  Port=2
  f : TriggerPort  TriggerType=function-call  VariantControl=Variant  StatesWhenEnabling=reset
      settings: CopyFcn=Stateflow.SLINSF.SimulinkMan.removeBlockPreDeleteFcn  PreDeleteFcn=Stateflow.SLINSF.SimulinkMan.unsafePredeleteFcn
  Calculate Downshift Threshold : Lookup_n-D  BreakpointsForDimension1=Pedal_Positions  BreakpointsForDimension2=2:8  Table=Downshift_Speeds  ExtrapMethod=Clip  UseLastTableValue=on  InternalRulePriority=Speed  RndMeth=Simplest  InputSameDT=on
  down_th : Outport
  wires:
  Calculate Downshift Threshold/1 -> down_th/1
  gear/1 -> Calculate Downshift Threshold/2
  pedal/1 -> Calculate Downshift Threshold/1

== system Copy_of_MPC_control/all_system/Controllers1/Transmission Controller/TCM/TCM Shift Controller/calc_up ==
  gear : Inport
  pedal : Inport  Port=2
  f : TriggerPort  TriggerType=function-call  VariantControl=Variant  StatesWhenEnabling=reset
      settings: CopyFcn=Stateflow.SLINSF.SimulinkMan.removeBlockPreDeleteFcn  PreDeleteFcn=Stateflow.SLINSF.SimulinkMan.unsafePredeleteFcn
  Calculate Upshift Threshold : Lookup_n-D  BreakpointsForDimension1=Pedal_Positions  BreakpointsForDimension2=1:7  Table=Upshift_Speeds  ExtrapMethod=Clip  UseLastTableValue=on  InternalRulePriority=Speed  RndMeth=Simplest  InputSameDT=on
  up_th : Outport
  wires:
  Calculate Upshift Threshold/1 -> up_th/1
  pedal/1 -> Calculate Upshift Threshold/1
  gear/1 -> Calculate Upshift Threshold/2

== system Copy_of_MPC_control/all_system/Visualization1/3D Engine/3D Engine/Part Rotation Concatenation ==
  Body Roll : Inport
  Body Ptich : Inport  Port=2
  Body Yaw : Inport  Port=3
  WheelFrontLeft Pitch : Inport  Port=4
  WheelFrontRight Pitch : Inport  Port=5
  WheelRearLeft Pitch : Inport  Port=6
  WheelRearRight Ptich : Inport  Port=7
  WheelFrontLeft Roll : Inport  Port=8
  WheelFrontRight Roll : Inport  Port=9
  WheelRearLeft Roll : Inport  Port=10
  WheelRearRight Roll : Inport  Port=11
  WheelFrontLeft Yaw : Inport  Port=12
  WheelFrontRight Yaw : Inport  Port=13
  WheelRearLeft Yaw : Inport  Port=14
  WheelRearRight Yaw : Inport  Port=15
  AllParts : Concatenate  NumInputs=5  Mode=Multidimensional array
  Body : Concatenate  NumInputs=3  Mode=Multidimensional array  ConcatenateDimension=2
  WheelFrontLeft : Concatenate  NumInputs=3  Mode=Multidimensional array  ConcatenateDimension=2
  WheelFrontRight : Concatenate  NumInputs=3  Mode=Multidimensional array  ConcatenateDimension=2
  WheelRearLeft : Concatenate  NumInputs=3  Mode=Multidimensional array  ConcatenateDimension=2
  WheelRearRight : Concatenate  NumInputs=3  Mode=Multidimensional array  ConcatenateDimension=2
  ConcatOut : Outport
  wires:
  Body Ptich/1 -> Body/1
  Body Yaw/1 -> Body/3
  WheelFrontLeft Pitch/1 -> WheelFrontLeft/1
  WheelFrontLeft Yaw/1 -> WheelFrontLeft/3
  WheelFrontLeft Roll/1 -> WheelFrontLeft/2
  Body Roll/1 -> Body/2
  WheelFrontLeft/1 -> AllParts/2
  WheelRearRight Ptich/1 -> WheelRearRight/1
  Body/1 -> AllParts/1
  WheelRearLeft/1 -> AllParts/4
  WheelFrontRight/1 -> AllParts/3
  WheelRearRight Yaw/1 -> WheelRearRight/3
  WheelFrontRight Roll/1 -> WheelFrontRight/2
  WheelFrontRight Pitch/1 -> WheelFrontRight/1
  WheelRearRight Roll/1 -> WheelRearRight/2
  WheelRearLeft Yaw/1 -> WheelRearLeft/3
  AllParts/1 -> ConcatOut/1
  WheelRearLeft Roll/1 -> WheelRearLeft/2
  WheelRearRight/1 -> AllParts/5
  WheelRearLeft Pitch/1 -> WheelRearLeft/1
  WheelFrontRight Yaw/1 -> WheelFrontRight/3

== system Copy_of_MPC_control/all_system/Visualization1/3D Engine/3D Engine/Part Translation Concatenation ==
  BodyX : Inport
  BodyY : Inport  Port=2
  BodyZ : Inport  Port=3
  WheelFrontLeftX : Inport  Port=4
  WheelFrontRightX : Inport  Port=5
  WheelRearLeftX : Inport  Port=6
  WheelRearRightX : Inport  Port=7
  WheelFrontLeftY : Inport  Port=8
  WheelFrontRightY : Inport  Port=9
  WheelRearLeftY : Inport  Port=10
  WheelRearRightY : Inport  Port=11
  WheelFrontLeftZ : Inport  Port=12
  WheelFrontRightZ : Inport  Port=13
  WheelRearLeftZ : Inport  Port=14
  WheelRearRightZ : Inport  Port=15
  AllParts : Concatenate  NumInputs=5  Mode=Multidimensional array
  Body : Concatenate  NumInputs=3  Mode=Multidimensional array  ConcatenateDimension=2
  WheelFrontLeft : Concatenate  NumInputs=3  Mode=Multidimensional array  ConcatenateDimension=2
  WheelFrontRight : Concatenate  NumInputs=3  Mode=Multidimensional array  ConcatenateDimension=2
  WheelRearLeft : Concatenate  NumInputs=3  Mode=Multidimensional array  ConcatenateDimension=2
  WheelRearRight : Concatenate  NumInputs=3  Mode=Multidimensional array  ConcatenateDimension=2
  ConcatOut : Outport
  wires:
  BodyX/1 -> Body/1
  BodyZ/1 -> Body/3
  WheelFrontLeftX/1 -> WheelFrontLeft/1
  WheelFrontLeftZ/1 -> WheelFrontLeft/3
  WheelFrontLeftY/1 -> WheelFrontLeft/2
  BodyY/1 -> Body/2
  WheelFrontLeft/1 -> AllParts/2
  WheelRearRightX/1 -> WheelRearRight/1
  Body/1 -> AllParts/1
  WheelRearLeft/1 -> AllParts/4
  WheelFrontRight/1 -> AllParts/3
  WheelRearRightZ/1 -> WheelRearRight/3
  WheelFrontRightY/1 -> WheelFrontRight/2
  WheelFrontRightX/1 -> WheelFrontRight/1
  WheelRearRightY/1 -> WheelRearRight/2
  WheelRearLeftZ/1 -> WheelRearLeft/3
  AllParts/1 -> ConcatOut/1
  WheelRearLeftY/1 -> WheelRearLeft/2
  WheelRearRight/1 -> AllParts/5
  WheelRearLeftX/1 -> WheelRearLeft/1
  WheelFrontRightZ/1 -> WheelFrontRight/3

== system Copy_of_MPC_control/all_system/Visualization1/3D Engine/3D Engine/Scale ==
  Constant{1..12,17,32..33} (15 alike) : Constant  OutDataTypeStr=single
  PartConcatenation : Subsystem
  ScaleOut : Outport
  wires:
  Constant10/1 -> PartConcatenation/15(WheelRearRightZ)
  Constant9/1 -> PartConcatenation/14(WheelRearRightY)
  Constant11/1 -> PartConcatenation/13(WheelRearRightX)
  Constant7/1 -> PartConcatenation/12(WheelRearLeftZ)
  Constant6/1 -> PartConcatenation/11(WheelRearLeftY)
  Constant8/1 -> PartConcatenation/10(WheelRearLeftX)
  Constant4/1 -> PartConcatenation/9(WheelFrontRightZ)
  Constant3/1 -> PartConcatenation/8(WheelFrontRightY)
  Constant5/1 -> PartConcatenation/7(WheelFrontRightX)
  Constant2/1 -> PartConcatenation/6(WheelFrontLeftZ)
  Constant1/1 -> PartConcatenation/5(WheelFrontLeftY)
  Constant33/1 -> PartConcatenation/4(WheelFrontLeftX)
  Constant32/1 -> PartConcatenation/3(BodyZ)
  Constant17/1 -> PartConcatenation/2(BodyY)
  Constant12/1 -> PartConcatenation/1(BodyX)
  PartConcatenation/1(ConcatOut) -> ScaleOut/1

== system Copy_of_MPC_control/all_system/Controllers1/Brake Controller/Brake Pressure Control/Bang Bang ABS/Bang-bang controller ==
  in_1 : Inport
  Constant : Constant  Value=0
  Data Type Conversion1 : DataTypeConversion  OutDataTypeStr=double  SaturateOnIntegerOverflow=on  RndMeth=Zero
  Data Type Conversion2 : DataTypeConversion  OutDataTypeStr=double  SaturateOnIntegerOverflow=on  RndMeth=Zero
  Relational Operator : RelationalOperator  Operator=>  OutDataTypeStr=boolean  RndMeth=Nearest  InputSameDT=on
  Relational Operator1 : RelationalOperator  Operator=<  OutDataTypeStr=boolean  RndMeth=Nearest  InputSameDT=on
  Sum : Sum  Inputs=+-  SaturateOnIntegerOverflow=on  InputSameDT=on  OutDataTypeStr=Inherit: Same as first input
  out_1 : Outport  InitialOutput=0
  wires:
  Data Type Conversion2/1 -> Sum/2
  Data Type Conversion1/1 -> Sum/1
  Sum/1 -> out_1/1
  Relational Operator/1 -> Data Type Conversion1/1
  Relational Operator1/1 -> Data Type Conversion2/1
  Constant/1 -> Relational Operator/2, Relational Operator1/2
  in_1/1 -> Relational Operator1/1, Relational Operator/1

== system Copy_of_MPC_control/all_system/Visualization1/3D Engine/3D Engine/Scale/PartConcatenation ==
  BodyX : Inport
  BodyY : Inport  Port=2
  BodyZ : Inport  Port=3
  WheelFrontLeftX : Inport  Port=4
  WheelFrontLeftY : Inport  Port=5
  WheelFrontLeftZ : Inport  Port=6
  WheelFrontRightX : Inport  Port=7
  WheelFrontRightY : Inport  Port=8
  WheelFrontRightZ : Inport  Port=9
  WheelRearLeftX : Inport  Port=10
  WheelRearLeftY : Inport  Port=11
  WheelRearLeftZ : Inport  Port=12
  WheelRearRightX : Inport  Port=13
  WheelRearRightY : Inport  Port=14
  WheelRearRightZ : Inport  Port=15
  AllParts : Concatenate  NumInputs=5  Mode=Multidimensional array
  Body : Concatenate  NumInputs=3  Mode=Multidimensional array  ConcatenateDimension=2
  WheelFrontLeft : Concatenate  NumInputs=3  Mode=Multidimensional array  ConcatenateDimension=2
  WheelFrontRight : Concatenate  NumInputs=3  Mode=Multidimensional array  ConcatenateDimension=2
  WheelRearLeft : Concatenate  NumInputs=3  Mode=Multidimensional array  ConcatenateDimension=2
  WheelRearRight : Concatenate  NumInputs=3  Mode=Multidimensional array  ConcatenateDimension=2
  ConcatOut : Outport
  wires:
  BodyX/1 -> Body/1
  BodyZ/1 -> Body/3
  WheelFrontLeftX/1 -> WheelFrontLeft/1
  WheelFrontLeftZ/1 -> WheelFrontLeft/3
  WheelFrontLeftY/1 -> WheelFrontLeft/2
  BodyY/1 -> Body/2
  WheelFrontLeft/1 -> AllParts/2
  WheelRearRightX/1 -> WheelRearRight/1
  Body/1 -> AllParts/1
  WheelRearLeft/1 -> AllParts/4
  WheelFrontRight/1 -> AllParts/3
  WheelRearRightZ/1 -> WheelRearRight/3
  WheelFrontRightY/1 -> WheelFrontRight/2
  WheelFrontRightX/1 -> WheelFrontRight/1
  WheelRearRightY/1 -> WheelRearRight/2
  WheelRearLeftZ/1 -> WheelRearLeft/3
  AllParts/1 -> ConcatOut/1
  WheelRearLeftY/1 -> WheelRearLeft/2
  WheelRearRight/1 -> AllParts/5
  WheelRearLeftX/1 -> WheelRearLeft/1
  WheelFrontRightZ/1 -> WheelFrontRight/3

== stateflow chart Copy_of_MPC_control/Controllers/Transmission Controller/TCM/TCM Shift Controller ==
  settings: sampleTime=0.01
  state GearState [parallel]
    settings: executionOrder=1
    state Neutral
      en:
      GearState = 0;
    state G1
      en:
      GearState = 1;
    state G2
      en:
      GearState = 2;
      du:
      [SpdThr] = calc(2,pedal,speed);
    state G3
      en:
      GearState = 3;
      du:
      [SpdThr] = calc(3,pedal,speed);
    state G8
      en:
      GearState = 8;
    state G7
      en:
      GearState = 7;
    state G6
      en:
      GearState = 6;
    state G5
      en:GearState=5;
      du:[SpdThr]=calc(5,pedal,speed);
    state G4
      en:
      GearState = 4;
      du:
      [SpdThr] = calc(4,pedal,speed);
    (default) -> G1
    Neutral -> G1 : [~Neutral]
    G1 -> G2 [order 1] : Up
    G2 -> G3 [order 1] : Up
    G1 -> Neutral [order 2] : [Neutral]
    G2 -> G1 [order 2] : Down
    G3 -> G2 [order 2] : Down
    G3 -> G4 [order 1] : Up
    G4 -> G3 [order 2] : Down
    G7 -> G8 [order 1] : Up
    G5 -> G6 [order 1] : Up
    G6 -> G7 [order 1] : Up
    G4 -> G5 [order 1] : Up
    G5 -> G4 [order 2] : Down
    G6 -> G5 [order 2] : Down
    G7 -> G6 [order 2] : Down
    G8 -> G7 : Down
  state SelectionState [parallel]
    du:[up_th]=calc_up(GearState,pedal);
    du:[down_th]=calc_down(GearState,pedal);
    settings: executionOrder=2
    state SteadyState
      en:
      clutchControl = 0;
    state preDownShifting
    state preUpShifting
    state UpShifting
      en:
      GearState = GearState + 0.5;
    state DownShifting
      en:
      GearState = GearState - 0.5;
    (default) -> SteadyState
    SteadyState -> (junction 62) [order 1] : [speed < down_th && ...
        | GearState >1]
    SteadyState -> (junction 128) [order 2] : [speed > up_th &&...
        | GearState <= 5 && ...
        | floor(GearState) == GearState]
    (junction 62) -> preDownShifting
    (junction 128) -> preUpShifting
    (junction 168) -> SteadyState
    (junction 23) -> SteadyState
    (junction 161) -> SteadyState
    preDownShifting -> (junction 168) [order 2] : [speed >= down_th]
    preUpShifting -> (junction 161) [order 2] : [speed <= up_th]
    preUpShifting -> UpShifting [order 1] : after(0.5,sec)
        | [speed>up_th]
    preDownShifting -> DownShifting [order 1] : after(0.5, sec)
        | [speed < down_th - 2]
    DownShifting -> (junction 23) : {GearState.Down;}
    UpShifting -> (junction 23) : {GearState.Up;}
  state up_th = calc_up(gear,pedal) [function]
  state down_th = calc_down(gear,pedal) [function]
  state SpdThr = calc(gear,pedal,speed) [function]
  data: gear function_input; pedal function_input; up_th function_output; gear function_input; pedal function_input; down_th function_output; gear function_input; pedal function_input; SpdThr function_output; speed function_input; GearState output int8; speed input; pedal input; clutchControl local double; SpdThr local double; Neutral input; up_th local double; down_th local double
  events: Up local EITHER_EDGE_EVENT; Down local EITHER_EDGE_EVENT

== matlab function Copy_of_MPC_control/Mpc_block/Mpc ==
  data: lambda output; r output; JE input; JF_part input; Fxh input; M input; Np input; U_min input; U_max input; Heading_updated input [1..5]; Velocity_updated input [1..5]; Rs input; Tsim input; U_delay input; U output
function [lambda, r, U] = HQP_solver(JE, JF_part, Fxh, M, Np, U_min, U_max, Heading_updated, Velocity_updated, Rs, Tsim, U_delay)
U = zeros(2,1);
du1_inc = 1*5/3*pi;du1_dec = 1*5/3*pi;
du2_inc = 1;du2_dec = 1;
dU_plus = []; dU_minus = [];
for i = 1:Np
    dU_plus = [dU_plus; [U_delay(1) + du1_inc; U_delay(2) + du2_inc]];
    dU_minus = [dU_minus; [-U_delay(1) + du1_dec; -U_delay(2) + du2_dec;]];
end
N = [U_max;
      U_min;
      dU_plus;
      dU_minus;          
     ];
if Tsim > 0
    for i = 1: Np
        Rs(2*i,:) = Heading_updated(i,:);
        Rs(2*i-1,:) = Velocity_updated(i,:);
    end
end
JF = JF_part*(Rs-Fxh);
[u,lambda]= HQP(JE,JF,M,N);
U = u(1:2);
r = Rs(1:2,:);
end

== matlab function Copy_of_MPC_control/MATLAB Function ==
  data: u input; Ac output; Br output
function [Ac, Br] = choose(u)
Ac = 0; Br = 0;
if u > 0 || u == 0
    Ac = u;
else
    Br = abs(u);
end
end

== matlab function Copy_of_MPC_control/observer/observer_1/gate ==
  data: select_overlap input; state output
function state = gate(select_overlap)
if select_overlap == 1
    state = 1;
else
    state = 0;
end
end

== matlab function Copy_of_MPC_control/observer/simulator_1/Mpc_Simulator_Middle/MATLAB Function ==
  data: r output; JE input; phi input; Fxh input; Qc input; U output; M input; Np input; Heading_updated input; Velocity_updated input; Rs input; Tsim input; select_MPC input; U_delay input
function [r,U] = HQP(JE ,phi,Fxh ,Qc ,M ,Np,Heading_updated ,Velocity_updated ,Rs ,Tsim, select_MPC,U_delay)
u1_max =  5/3*pi; u1_min = -5/3*pi;
u2_max =  1; u2_min = -1;
du1_inc =  1*5/3*pi;du1_dec =  1*5/3*pi;
du2_inc =  1;du2_dec =  1;
U_max = []; U_min = [];
for i = 1:Np
    U_max = [U_max; [u1_max; u2_max]];
    U_min = [U_min; [-u1_min; -u2_min]];
end

dU_plus = []; dU_minus = [];
for i = 1:Np
    dU_plus = [dU_plus; [U_delay(1) + du1_inc; U_delay(2) + du2_inc]];
    dU_minus = [dU_minus; [-U_delay(1) + du1_dec; -U_delay(2) + du2_dec;]];
end
N = [U_max;
      U_min;
      dU_plus;
      dU_minus;          
     ];
if Tsim > 0 && select_MPC ~= 5
    for i = 1: Np
        Rs(2*i,:) = Heading_updated(i,:);
        Rs(2*i-1,:) = Velocity_updated(i,:);
    end
end
JF = -2*phi'*Qc*(Rs-Fxh);
[u,lambda]= HQP(JE,JF,M,N);
U = u(1:2);
r = Rs(1:2,:);
end

== matlab function Copy_of_MPC_control/observer/simulator_3/Mpc_Simulator_Middle/MATLAB Function ==
  data: r output; JE input; phi input; Fxh input; Qc input; U output; M input; Np input; Heading_updated input; Velocity_updated input; Rs input; Tsim input; select_MPC input; U_delay input
function [r,U] = HQP(JE ,phi,Fxh ,Qc ,M ,Np,Heading_updated ,Velocity_updated ,Rs ,Tsim, select_MPC ,U_delay)
u1_max =  5/3*pi; u1_min = -5/3*pi;
u2_max =  1; u2_min = -1;
du1_inc =  1*5/3*pi;du1_dec =  1*5/3*pi;
du2_inc =  1;du2_dec =  1;
U_max = []; U_min = [];
for i = 1:Np
    U_max = [U_max; [u1_max; u2_max]];
    U_min = [U_min; [-u1_min; -u2_min]];
end

dU_plus = []; dU_minus = [];
for i = 1:Np
    dU_plus = [dU_plus; [U_delay(1) + du1_inc; U_delay(2) + du2_inc]];
    dU_minus = [dU_minus; [-U_delay(1) + du1_dec; -U_delay(2) + du2_dec;]];
end
N = [U_max;
      U_min;
      dU_plus;
      dU_minus;          
     ];
if Tsim > 0 && select_MPC ~= 5
    for i = 1: Np
        Rs(2*i,:) = Heading_updated(i,:);
        Rs(2*i-1,:) = Velocity_updated(i,:);
    end
end
JF = -2*phi'*Qc*(Rs-Fxh);
[u,lambda]= HQP(JE,JF,M,N);
U = u(1:2);
r = Rs(1:2,:);
end

== matlab function Copy_of_MPC_control/Passenger Vehicle/beta ==
  data: xdot input; beta output; ydot input; Velocity output
function [beta, Velocity]  = Velocity_Beta(xdot, ydot)
beta = 0; Velocity = 0;
Velocity = sqrt(xdot^2 + ydot^2);
xdot = abs(xdot);
beta = atan2(ydot, xdot);
end
